simulink model "amk_sim_model"  (R2022b)
settings: Solver=FixedStepAuto  StartTime=0.0  StopTime=4  FixedStep=1e-6  MaxStep=1e-5  MinStep=1e-6  RelTol=1e-3
values from neighbouring files (symbols this model uses):
  a_fw = log(9)/trfw    [amk_sim.m]    (also in amk_sim_2.m)
  ac = log(9)/tr    [amk_sim.m]    (also in amk_sim_2.m)
  ar_max = 1500    [amk_sim_2.m]
  as = log(9)/trs    [amk_sim.m]    (also in amk_sim_2.m)
  ba = 2*k^2*(as*J - 0)/(np^2*psi)    [amk_sim.m]    (also in amk_sim_2.m = 2*k^2*(as*J - bm)/(np^2*psi))
  bm = 0.02    [amk_sim.m]    (also in amk_sim_2.m = 0.008)
  I_base = 85.7    [amk_sim.m]    (also in amk_sim_2.m)
  I_max = 85.7    [amk_sim.m]    (also in amk_sim_2.m)
  Icon = 33.5    [amk_sim.m]    (also in amk_sim_2.m)
  Imax_interval = 1.24    [amk_sim.m]    (also in amk_sim_2.m = 5)
  Ipeak = 85.7    [amk_sim.m]    (also in amk_sim_2.m = 87.5)
  J = 2.5*(2.74e-4)    (= 0.000685)    [amk_sim.m]    (also in amk_sim_2.m = 0.000528)
  k = 1    [amk_sim.m]    (also in amk_sim_2.m)
  ki_ar = 0.2    [amk_sim_2.m]
  ki_s = 2*k^2*as^2*J/(np^2*psi)    [amk_sim.m]    (also in amk_sim_2.m)
  kp_ar = 1e-5    (= 1e-05)    [amk_sim_2.m]
  kp_s = 2*k^2*as*J/(np^2*psi)    [amk_sim.m]    (also in amk_sim_2.m)
  Ld = Ldm    (= 0.0004)    [amk_sim.m]    (also in amk_sim_2.m = 0.00012)
  Lq = Lqm    (= 0.00052)    [amk_sim.m]    (also in amk_sim_2.m = 0.00024)
  max_temp = 140    [amk_sim.m]    (also in amk_sim_2.m)
  np = 5    [amk_sim.m]    (also in amk_sim_2.m)
  Peak_power = 45000    [amk_sim.m]    (also in amk_sim_2.m = 50000)
  Peak_regen = -15000    [amk_sim.m]    (also in amk_sim_2.m = -1500000)
  psi = 0.047    [amk_sim.m]    (also in amk_sim_2.m = 0.05077789)
  rpm_nom = 20000    [amk_sim.m]    (also in amk_sim_2.m = 12000)
  Rs = 202.5e-3    (= 0.2025)    [amk_sim.m]    (also in amk_sim_2.m)
  sample_time = 1e-4    (= 0.0001)    [amk_sim.m]    (also in amk_sim_2.m = 1e-06)
  temp_threshold = 100    [amk_sim.m]    (also in amk_sim_2.m)
  u_dc = 550    [amk_sim.m]    (also in amk_sim_2.m)
  u_nom = u_dc*k    (= 550)    [amk_sim.m]    (also in amk_sim_2.m)
undefined symbols (not defined in the file or in its folder): sigbuilder_block
libraries: simulink x3
(part 1 of 5)
settings Model: Creator=Vaggelis  LastModifiedBy=alexa
settings SolverCC: ZeroCrossAlgorithm=Adaptive
settings OptimizationCC: ReuseModelBlockBuffer=on
settings DebuggingCC: IgnoredZcDiagnostic=none  UnconnectedInputMsg=warning  UnconnectedOutputMsg=warning  UnconnectedLineMsg=warning  ArithmeticOperatorsInVariantConditions=warning
settings ModelReferenceCC: EnableRefExpFcnMdlSchedulingChecks=on  ModelReferenceMinAlgLoopOccurrences=on
settings SFSimCC: CustomCodeUndefinedFunction=UseInterfaceOnly
settings RTWCC: DLArmComputeVersion=19.05

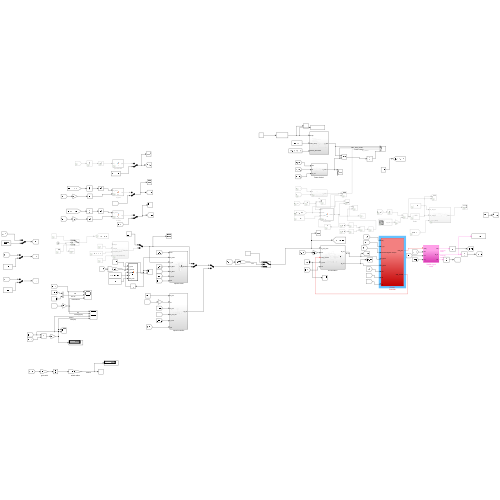
[thumbnail: Simulink's stored preview of the top-level diagram]
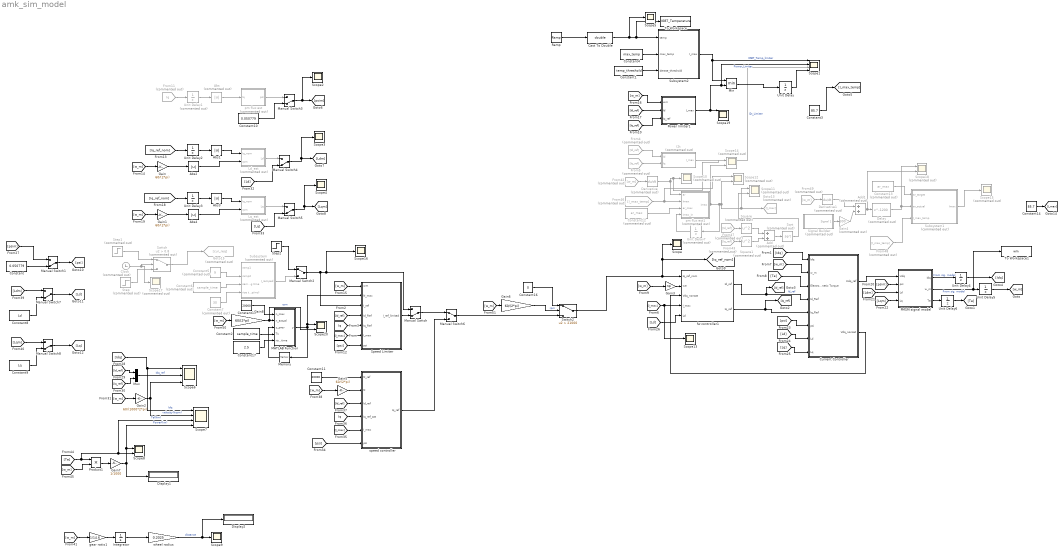
== system amk_sim_model ==
  Abs : Abs  Commented=on  SaturateOnIntegerOverflow=off
  Abs{1..4} (4 alike) : Abs  SaturateOnIntegerOverflow=off
  Add : Sum  Commented=on
  Add1 : Sum  Commented=on
  Cast To Double : DataTypeConversion  OutDataTypeStr=double  SaturateOnIntegerOverflow=off  RndMeth=Floor
  Clock : Clock  Commented=on
  Constant : Constant  Value=0.050779
  Constant1 : Constant  Value=temp_threshold
  Constant10 : Constant  Value=0.050779
  Constant11 : Constant  Value=20000
  Constant12 : Constant  Commented=on  Value=ar_max
  Constant13 : Constant  Commented=on  Value=ar_max
  Constant14 : Constant  Value=85.7
  Constant15 : Constant  Value=20000
  Constant16 : Constant  Value=0
  Constant17 : Constant  Value=2.5
  Constant2 : Constant  Value=sample_time
  Constant3 : Constant  Value=85.7
  Constant4 : Constant  Value=max_temp
  Constant5 : Constant  Commented=on  Value=9
  Constant6 : Constant  Commented=on  Value=sample_time
  Constant7 : Constant  Commented=on  Value=30
  Constant8 : Constant  Value=Ld
  Constant9 : Constant  Value=Lq
  Current Controller : Subsystem
  Delay : Delay  Commented=on  DelayLength=1200  InitialCondition=0  UseCircularBuffer=on
  Derivative : Derivative  Commented=on
  Derivative1 : Derivative  Commented=on
  Display1 : Display
  Display2 : Display
  From11 : From  Commented=on  GotoTag=Iq  TagVisibility=global
  From4 : From  Commented=on  GotoTag=Id_ref
  From42 : From  Commented=on  GotoTag=w_m
  From43 : From  Commented=on  GotoTag=Iq_ref
  From46 : From  Commented=on  GotoTag=I_max_temp
  From47 : From  Commented=on  GotoTag=Id_ref
  From48 : From  Commented=on  GotoTag=I_max_temp
  From49 : From  Commented=on  GotoTag=w_m
  From5 : From  Commented=on  GotoTag=Iq_ref
  Gain{,1,5..6,8} (5 alike) : Gain  Gain=60/(2*pi)
  Gain2 : Gain  Gain=60/(1000*2*pi)
  Gain3 : Gain  Gain=np
  Gain4 : Gain  Commented=on  Gain=300
  Gain7 : Gain  Gain=1/1000
  Goto13 : Goto  Commented=on  GotoTag=I_max
  Goto15 : Goto  Commented=on  GotoTag=cur_req
  I2t : Subsystem  Commented=on
  Integrator : Integrator
  Ld_est : MATLAB Function  Commented=on  TreatAsAtomicUnit=on
  Lq_est : MATLAB Function  Commented=on  TreatAsAtomicUnit=on
  MATLAB Function : MATLAB Function  TreatAsAtomicUnit=on
  Manual Switch{,1,3..5,7..8} (7 alike) : ManualSwitch  CurrentSetting=0
  Manual Switch2 : ManualSwitch
  Manual Switch6 : ManualSwitch
  Memory : Memory
  Min : MinMax  Inputs=2
  Mux : Mux  Inputs=2
  PMSM signal model : Subsystem
  Power limiter1 : Subsystem
  Product1 : Product
  Ramp : simulink/Sources/Ramp  slope=1  start=0  InitialOutput=30
  Scope{,2..5,9,13,16} (8 alike) : Scope
  Scope1 : Scope  NumInputPorts=4
  Scope10 : Scope  Commented=on
  Scope{11..12,14,18} (4 alike) : Scope  Commented=on  NumInputPorts=2
  Scope15 : Scope  Commented=on
  Scope17 : Scope  Commented=on
  Scope19 : Scope  NumInputPorts=4
  Scope20 : Scope  NumInputPorts=2
  Scope6 : Scope  NumInputPorts=3
  Scope7 : Scope  NumInputPorts=4
  Scope8 : Scope  NumInputPorts=2
  Signal Builder : Subsystem  Tag=STV Subsys  Commented=on  LoadFcn=sigbuilder_block('load');  StartFcn=sigbuilder_block('start');  StopFcn=sigbuilder_block('stop');  ClipboardFcn=sigbuilder_block('clipboard');  mask(Sigbuilder block){tuvar=[0:10]}
      mask help: Simulink:masks:SigbuilderBlock_MD
      mask init:
      | if ~strcmp(get_param(bdroot(gcbh),'SimulationStatus'),'stopped') tuvar = sigbuilder_block('maskInit'); end
      settings: CopyFcn=sigbuilder_block('copy');  DeleteFcn=sigbuilder_block('delete');  ModelCloseFcn=sigbuilder_block('modelClose');  PreSaveFcn=sigbuilder_block('preSave');  PauseFcn=sigbuilder_block('pause');  ContinueFcn=sigbuilder_block('continue');  NameChangeFcn=sigbuilder_block('namechange');  OpenFcn=sigbuilder_block('open',[437.6 199.2 550.4 400 ]);  CloseFcn=sigbuilder_block('close');
      mask Display: plot(0, 0, 100, 100,[2, 2, 32, 32, 2], [68, 8, 8, 68, 68],[32, 2], [38, 38], [32, 19, 2],[53, 60, 44], [32, 17, 17, 2],[16, 16, 31, 31]);txt = getActiveGroup(gcbh);text(2, 100, txt,'verticalAlignment', 'top');
  Speed Limiter : Subsystem
  Sqrt : Sqrt  Commented=on
  Square : Math  Commented=on  Operator=square
  Square1 : Math  Commented=on  Operator=square
  Step : Step  Commented=on  Time=0.3  After=90  SampleTime=0
  Step1 : Step  Commented=on  After=90  SampleTime=0
  Step2 : Step  Time=0.5  Before=90  After=90  SampleTime=0
  Subsystem : Subsystem  Commented=on
  Subsystem1 : Subsystem  Commented=on
  Subsystem2 : Subsystem
  Switch : Switch  Commented=on  Criteria=u2 > Threshold  Threshold=0.8  SaturateOnIntegerOverflow=off  InputSameDT=off
  Switch2 : Switch  Criteria=u2 > Threshold  Threshold=21000  SaturateOnIntegerOverflow=off  InputSameDT=off
  To Workspace : ToWorkspace  VariableName=IGBT_Temperature  SampleTime=-1
  To Workspace1 : ToWorkspace  VariableName=wm  SampleTime=-1
  Unit Delay{,2..6} (6 alike) : UnitDelay  SampleTime=-1  HasFrameUpgradeWarning=on
  Unit Delay1 : UnitDelay  Commented=on  SampleTime=-1  HasFrameUpgradeWarning=on
  Unit Delay7 : UnitDelay  Commented=on  SampleTime=-1  HasFrameUpgradeWarning=on
  fw controller1 : Subsystem
  gear ratio1 : Gain  Gain=1/14.6
  pm flux est : MATLAB Function  Commented=on  TreatAsAtomicUnit=on
  pm flux est1 : MATLAB Function  Commented=on  TreatAsAtomicUnit=on
  speed controller : Subsystem
  wheel radius : Gain  Gain=0.2025
  wires:
  PMSM signal model/2("w_m ") -> To Workspace1/1, Unit Delay5/1  "From sig. model"
  Gain3/1 -> fw controller1/2(we)
  Current Controller/2(Vdq_nonsat) -> fw controller1/3(Vdq_nonsat)
  PMSM signal model/1(Idq) -> Unit Delay4/1  "From sig. model"
  [Idq] -> Current Controller/1(Idq)
  [w_m] -> Current Controller/2(w_m)
  [Te] -> Current Controller/3(Electromagnetic Torque)
  [w_m] -> Power limiter1/1(wm)
  [Id_ref] -> Power limiter1/2(Id)
  Current Controller/1("Udq_ref ") -> PMSM signal model/1(Udq)
  Constant5/1 -> Subsystem/2(ramp2)
  Constant6/1 -> Subsystem/3(sampling time)
  Constant7/1 -> Subsystem/4(rise time (Amp/ms))
  Constant4/1 -> Subsystem2/2(max_temp)
  Ramp/1 -> Cast To Double/1
  Cast To Double/1 -> Subsystem2/1(temp), To Workspace/1, Scope5/1
  fw controller1/1(Id_ref) -> Current Controller/4(Id_Ref), [Id_ref]  "Id_ref"
  From4/1 -> I2t/1(Id)
  From5/1 -> I2t/2(Iq)
  Subsystem2/1(I_max) -> Min/1, Scope1/1  "IGBT_Temp_limiter"
  Power limiter1/1(I_max) -> Scope1/2, Min/2, Scope19/1  "Power_Limiter"
  I2t/1(I_max) -> Scope1/3  "I2t_Limiter"
  [I_max] -> Speed Limiter/6(I_max)
  Unit Delay/1 -> Scope1/4
  [Iq_ref] -> Power limiter1/3(Iq_ref)
  Constant1/1 -> Subsystem2/3(derate_threshold)
  [I_max] -> Scope13/1, fw controller1/4(I_max)
  [Id_ref] -> Speed Limiter/4(Id_Ref)
  [Iq] -> Speed Limiter/5(Iq_Ref)
  [w_m] -> Speed Limiter/1(wm)
  [w_m] -> Gain3/1
  PMSM signal model/3("Te ") -> Unit Delay6/1
  Abs/1 -> pm flux est/1(Iq)
  From11/1 -> Unit Delay1/1
  [psi] -> Speed Limiter/7(psi)
  Unit Delay1/1 -> Abs/1
  Unit Delay2/1 -> Abs1/1
  [Iq_ref_nom] -> Unit Delay2/1
  Abs1/1 -> Ld_est/1(Iq_nom)
  [w_m] -> Gain/1
  Gain/1 -> Abs2/1
  Abs2/1 -> Ld_est/2(rpm)
  Abs4/1 -> Lq_est/2(rpm)
  Gain1/1 -> Abs4/1
  [w_m] -> Gain1/1
  Abs3/1 -> Lq_est/1(Iq_nom)
  [Iq_ref_nom] -> Unit Delay3/1
  Unit Delay3/1 -> Abs3/1
  [psim] -> PMSM signal model/2(psi)
  [Ldm] -> PMSM signal model/3(Ld)
  [Lqm] -> PMSM signal model/4(Lq)
  [psi] -> Current Controller/6(psi)
  [Ld] -> Current Controller/7(Ld)
  [Lq] -> Current Controller/8(Lq)
  [Ld] -> fw controller1/5(Ld)
  Speed Limiter/1(I_ref_limited) -> Manual Switch/2
  Unit Delay4/1 -> [Idq]
  Unit Delay5/1 -> [w_m]
  Unit Delay6/1 -> [Te]
  Manual Switch1/1 -> [psi]
  Constant/1 -> Manual Switch1/2
  [psim] -> Manual Switch1/1
  [Id_ref] -> Mux/1
  [Iq_ref] -> Mux/2
  Mux/1 -> Scope6/2  "Idq_ref"
  [Idq] -> Scope7/1, Scope6/1  "Idq"
  [w_m] -> Gain2/1
  Gain2/1 -> Scope6/3, Scope7/2  "velocity(krpm)"
  Subsystem/1(I_ramped) -> Manual Switch2/2
  Manual Switch2/1 -> Speed Limiter/3(I_ref), Scope16/1, Manual Switch/1
  pm flux est/1(psi) -> Manual Switch3/1
  Manual Switch3/1 -> Scope2/1, [psim]
  Constant10/1 -> Manual Switch3/2
  Ld_est/1(Ld) -> Manual Switch4/1
  Manual Switch4/1 -> [Ldm], Scope3/1
  [Ld] -> Manual Switch4/2
  Lq_est/1(Lq) -> Manual Switch5/1
  Manual Switch5/1 -> Scope4/1, [Lqm]
  [Lq] -> Manual Switch5/2
  speed controller/1(Iq_ref) -> Manual Switch6/2
  Constant11/1 -> speed controller/1(N_ref)
  [Iq] -> speed controller/4(Iq_ref_sat)
  [w_m] -> Gain5/1
  Gain5/1 -> speed controller/2(N)
  [Id_ref] -> speed controller/3(Id_ref)
  [psi] -> speed controller/6(psi)
  [I_max] -> speed controller/5(I_max)
  Manual Switch/1 -> Manual Switch6/1
  Manual Switch7/1 -> [Ld]
  Constant8/1 -> Manual Switch7/2
  Manual Switch8/1 -> [Lq]
  Constant9/1 -> Manual Switch8/2
  [Ldm] -> Manual Switch7/1
  [Lqm] -> Manual Switch8/1
  Gain7/1 -> Scope7/4, Scope8/1, Display1/1  "Power(kw)"
  Product1/1 -> Gain7/1
  [w_m] -> Product1/2
  [Te] -> Product1/1, Scope7/3, Scope8/2  "Te(Nm)"
  [w_m] -> gear ratio1/1
  Integrator/1 -> wheel radius/1
  wheel radius/1 -> Display2/1, Scope9/1  "distance"
  gear ratio1/1 -> Integrator/1
  Derivative/1 -> pm flux est1/1(ar), Scope14/1, Scope10/1
  From42/1 -> Derivative/1
  Min/1 -> Unit Delay/1
  From46/1 -> Scope12/1, pm flux est1/2(Imax)
  Constant12/1 -> pm flux est1/3(ar_max)
  Unit Delay7/1 -> pm flux est1/4(imax_in)
  From47/1 -> Square/1
  From43/1 -> Square1/1
  Square/1 -> Add/1
  Square1/1 -> Add/2
  Add/1 -> Sqrt/1
  Sqrt/1 -> Scope11/2
  pm flux est1/1(imax) -> Scope14/2, Unit Delay7/1, Scope12/2, Goto13/1, Scope11/1
  Constant13/1 -> Subsystem1/1(ar_target)
  From49/1 -> Derivative1/1
  Switch/1 -> Goto15/1
  Clock/1 -> Scope17/1, Switch/2
  Step/1 -> Switch/3
  Step1/1 -> Switch/1
  From48/1 -> Subsystem1/3(I_max_temp)
  Derivative1/1 -> Add1/1
  Signal Builder/1(Signal 1) -> Gain4/1
  Gain4/1 -> Add1/2
  Add1/1 -> Scope18/2, Delay/1
  Delay/1 -> Scope18/1, Subsystem1/2(ar_actual)
  Constant3/1 -> [I_max_temp]
  Step2/1 -> Manual Switch2/1
  Subsystem1/1(Imax) -> Scope15/1
  Constant14/1 -> [I_max]
  fw controller1/2(Iq_ref) -> [Iq_ref], Current Controller/5(Iq_Ref)
  Gain6/1 -> Switch2/2  "rpm"
  [w_m] -> Gain6/1
  Constant16/1 -> Switch2/1
  Manual Switch6/1 -> Switch2/3
  Switch2/1 -> Scope/1, [Iq_ref_nom], fw controller1/1(Iq_ref_nom)
  Constant15/1 -> MATLAB Function/1(n_max)
  MATLAB Function/1(y) -> Speed Limiter/2(N_max), Scope20/1, Memory/1
  Constant2/1 -> MATLAB Function/4(Ts)
  Constant17/1 -> MATLAB Function/5(rise_time)
  Memory/1 -> MATLAB Function/3(y_prev)
  [w_m] -> Gain8/1
  Gain8/1 -> Scope20/2, MATLAB Function/2(n_actual)  "rpm"

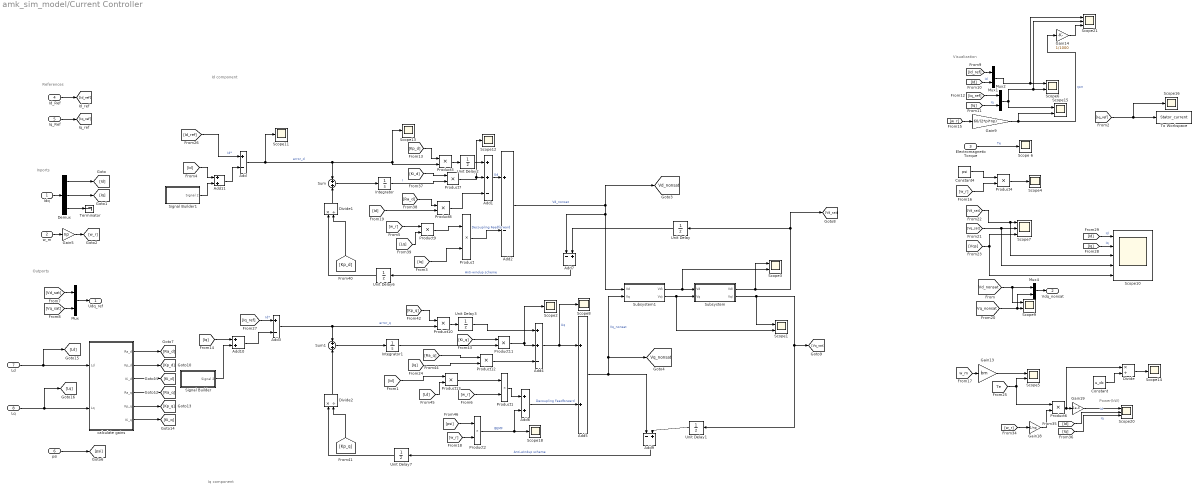
== system amk_sim_model/Current Controller ==
  note: References
  note: Id component
  note: Iq component
  note: Inports
  note: Outports
  note: Visualization
  note: Power(kW)
  Idq : Inport
  w_m : Inport  Port=2
  Electromagnetic Torque : Inport  Port=3
  Id_Ref : Inport  Port=4
  Iq_Ref : Inport  Port=5
  psi : Inport  Port=6
  Ld : Inport  Port=7
  Lq : Inport  Port=8
  Add : Sum  Inputs=+-
  Add1 : Sum  Inputs=++-
  Add{5..6,10..11} (4 alike) : Sum
  Add2 : Sum  Inputs=+-
  Add3 : Sum  Inputs=+-
  Add4 : Sum  Inputs=++-
  Add7 : Sum  Inputs=-+
  Add9 : Sum  Inputs=-+
  Constant : Constant  Value=u_dc
  Constant4 : Constant  Value=psi
  Demux : Demux  Outputs=3
  Divide : Product  Inputs=*/
  Divide1 : Product  Inputs=*/
  Divide2 : Product  Inputs=*/
  Gain13 : Gain  Gain=bm
  Gain14 : Gain  Gain=1/1000
  Gain18 : Gain  Gain=1/np
  Gain19 : Gain  Gain=1e-3
  Gain5 : Gain  Gain=np
  Gain9 : Gain  Gain=60/(2*pi*np)
  Integrator : Integrator
  Integrator1 : Integrator
  Mux{,1..2,4} (4 alike) : Mux  Inputs=2
  Product{,1..4,6..13} (13 alike) : Product
  Scope 6 : Scope
  Scope{1,3,5..6,9,15} (6 alike) : Scope  NumInputPorts=2
  Scope10 : Scope  NumInputPorts=5
  Scope{2,4,8,11..14,16,18} (9 alike) : Scope
  Scope20 : Scope  NumInputPorts=3
  Scope21 : Scope  NumInputPorts=3
  Scope7 : Scope  NumInputPorts=3
  Signal Builder : Subsystem  Tag=STV Subsys  LoadFcn=sigbuilder_block('load');  StartFcn=sigbuilder_block('start');  StopFcn=sigbuilder_block('stop');  ClipboardFcn=sigbuilder_block('clipboard');  mask(Sigbuilder block){tuvar=[0:10]}
      mask help: Simulink:masks:SigbuilderBlock_MD
      mask init:
      | if ~strcmp(get_param(bdroot(gcbh),'SimulationStatus'),'stopped') tuvar = sigbuilder_block('maskInit'); end
      settings: CopyFcn=sigbuilder_block('copy');  DeleteFcn=sigbuilder_block('delete');  ModelCloseFcn=sigbuilder_block('modelClose');  PreSaveFcn=sigbuilder_block('preSave');  PauseFcn=sigbuilder_block('pause');  ContinueFcn=sigbuilder_block('continue');  NameChangeFcn=sigbuilder_block('namechange');  OpenFcn=sigbuilder_block('open',[437.6 199.2 550.4 400 ]);  CloseFcn=sigbuilder_block('close');
      mask Display: plot(0, 0, 100, 100,[2, 2, 32, 32, 2], [68, 8, 8, 68, 68],[32, 2], [38, 38], [32, 19, 2],[53, 60, 44], [32, 17, 17, 2],[16, 16, 31, 31]);txt = getActiveGroup(gcbh);text(2, 100, txt,'verticalAlignment', 'top');
  Signal Builder1 : Subsystem  Tag=STV Subsys  LoadFcn=sigbuilder_block('load');  StartFcn=sigbuilder_block('start');  StopFcn=sigbuilder_block('stop');  ClipboardFcn=sigbuilder_block('clipboard');  mask(Sigbuilder block){tuvar=[0:10]}
      mask help: Simulink:masks:SigbuilderBlock_MD
      mask init:
      | if ~strcmp(get_param(bdroot(gcbh),'SimulationStatus'),'stopped') tuvar = sigbuilder_block('maskInit'); end
      settings: CopyFcn=sigbuilder_block('copy');  DeleteFcn=sigbuilder_block('delete');  ModelCloseFcn=sigbuilder_block('modelClose');  PreSaveFcn=sigbuilder_block('preSave');  PauseFcn=sigbuilder_block('pause');  ContinueFcn=sigbuilder_block('continue');  NameChangeFcn=sigbuilder_block('namechange');  OpenFcn=sigbuilder_block('open',[437.6 199.2 550.4 400 ]);  CloseFcn=sigbuilder_block('close');
      mask Display: plot(0, 0, 100, 100,[2, 2, 32, 32, 2], [68, 8, 8, 68, 68],[32, 2], [38, 38], [32, 19, 2],[53, 60, 44], [32, 17, 17, 2],[16, 16, 31, 31]);txt = getActiveGroup(gcbh);text(2, 100, txt,'verticalAlignment', 'top');
  Subsystem : Subsystem
  Subsystem1 : Subsystem
  Sum : Sum
  Sum1 : Sum
  Terminator : Terminator
  To Workspace : ToWorkspace  VariableName=Stator_current  SampleTime=-1
  Unit Delay{,1..3,6..7} (6 alike) : UnitDelay  SampleTime=-1  HasFrameUpgradeWarning=on
  calculate gains : Subsystem
  "Udq_ref " : Outport  VectorParamsAs1DForOutWhenUnconnected=off
  Vdq_nonsat : Outport  Port=2
  tag scope: Vd_nonsat=global, Vq_nonsat=global
  wires:
  Product11/1 -> Add4/2, Scope2/1
  Add4/1 -> Scope8/1, Add5/1  "Uq"
  Add1/1 -> Add2/1  "Ud"
  Product9/1 -> Product/1
  Product10/1 -> Unit Delay3/1
  Product3/1 -> Unit Delay2/1
  [w_r] -> Product1/2
  Product13/1 -> Product1/1
  Idq/1 -> Demux/1
  Product/1 -> Add2/2  "Decoupling Feedforward"
  Divide1/1 -> Sum/2
  Add2/1 -> [Vd_nonsat], Subsystem1/1(Vd), Add7/1  "Vd_nonsat"
  Add7/1 -> Unit Delay6/1  "Anti-windup scheme"
  Add5/1 -> Add9/1, Subsystem1/2(Vq), [Vq_nonsat]  "Vq_nonsat"
  Divide2/1 -> Sum1/2
  Add9/1 -> Unit Delay7/1  "Anti-windup scheme"
  Demux/1 -> [Id]
  Demux/2 -> [Iq]
  Demux/3 -> Terminator/1
  w_m/1 -> Gain5/1
  Gain5/1 -> [w_r]
  [Vd_sat] -> Mux/1
  [Vq_sat] -> Mux/2
  Mux/1 -> "Udq_ref "/1
  Mux1/1 -> Scope21/1, Scope6/1
  [Id_ref] -> Mux1/1
  [Id] -> Mux1/2  "Id"
  [Iq_ref] -> Mux2/1
  [Iq] -> Mux2/2  "Iq"
  [w_r] -> Gain9/1
  Gain9/1 -> Scope15/2, Gain14/1  "rpm"
  [psi] -> Product2/1
  Product1/1 -> Add6/1
  Add6/1 -> Add5/2  "Decoupling Feedforward"
  Add/1 -> Product3/2, Scope13/1, Sum/1, Scope11/1  "error_d"
  Add3/1 -> Product10/2, Sum1/1  "error_q"
  Product7/1 -> Scope12/1, Add1/2
  [Vd_nonsat] -> Scope9/1, Mux4/1
  [Vq_nonsat] -> Mux4/2, Scope9/2
  [Vd_sat] -> Scope10/3, Scope7/1
  [Vq_sat] -> Scope10/4, Scope7/2
  [Vqs] -> Scope7/3, Scope10/5
  [w_r] -> Product4/2
  Constant4/1 -> Product4/1
  Product4/1 -> Scope4/1
  Id_Ref/1 -> [Id_ref]
  Iq_Ref/1 -> [Iq_ref]
  Gain13/1 -> Scope5/1
  [Te] -> Product6/1, Scope5/2
  [w_m] -> Gain13/1
  Mux2/1 -> Scope21/2, Scope6/2, Scope15/1
  [Iq] -> Scope10/2  "Iq"
  [Id] -> Scope10/1  "Id"
  [Id_ref] -> Add/1  "Id*"
  [w_r] -> Product2/2
  Product2/1 -> Scope18/1, Add6/2  "BEMF"
  Mux4/1 -> Vdq_nonsat/1
  [Iq_ref] -> Add3/1  "Id*"
  Gain19/1 -> Scope20/1
  [Iq] -> Scope20/3  "Iq"
  [Id] -> Scope20/2  "Id"
  Gain18/1 -> Product6/2
  Product6/1 -> Divide/1, Gain19/1
  [w_r] -> Gain18/1
  Product12/1 -> Add4/3
  Product8/1 -> Add1/3
  Constant/1 -> Divide/2
  Divide/1 -> Scope14/1
  [Id] -> Product8/2
  [Iq] -> Product/2
  [Iq_ref] -> To Workspace/1, Scope16/1
  Electromagnetic Torque/1 -> Scope 6/1  "Te"
  Unit Delay/1 -> Add7/2
  Unit Delay1/1 -> Add9/2
  Gain14/1 -> Scope21/3
  [Kp_d] -> Product3/1
  Integrator/1 -> Product7/2  "I"
  [Ki_d] -> Product7/1
  [Ra_d] -> Product8/1
  [w_r] -> Product9/1
  [Lq] -> Product9/2
  [Kp_q] -> Product10/1
  [Ki_q] -> Product11/1
  Integrator1/1 -> Product11/2
  [Iq] -> Product12/2
  [Ra_q] -> Product12/1
  [Ld] -> Product13/2
  [Id] -> Product13/1
  Ld/1 -> [Ld], calculate gains/1(Ld)
  Lq/1 -> [Lq], calculate gains/2(Lq)
  psi/1 -> [psi]
  calculate gains/1(Ra_d) -> [Ra_d]
  calculate gains/2(Kp_d) -> [Kp_d]
  calculate gains/3(Ki_d) -> [Ki_d]
  calculate gains/4(Ra_q) -> [Ra_q]
  calculate gains/5(Kp_q) -> [Kp_q]
  calculate gains/6(Ki_q) -> [Ki_q]
  Unit Delay2/1 -> Add1/1
  Unit Delay3/1 -> Add4/1
  Sum/1 -> Integrator/1
  Sum1/1 -> Integrator1/1
  Unit Delay6/1 -> Divide1/1
  Unit Delay7/1 -> Divide2/1
  [Kp_d] -> Divide1/2
  [Kp_q] -> Divide2/2
  Signal Builder/1(Signal 2) -> Add10/2
  Signal Builder1/1(Signal 2) -> Add11/2
  Subsystem1/2(Vq\) -> Scope1/2, Subsystem/2(Vq)
  Subsystem1/1(Vd\) -> Scope3/2, Subsystem/1(Vd)
  Subsystem/1(Vd\) -> Scope3/1, [Vd_sat], Unit Delay/1
  Subsystem/2(Vq\) -> Scope1/1, Unit Delay1/1, [Vq_sat]
  [Iq] -> Add10/1
  Add10/1 -> Add3/2
  [Id] -> Add11/1
  Add11/1 -> Add/2

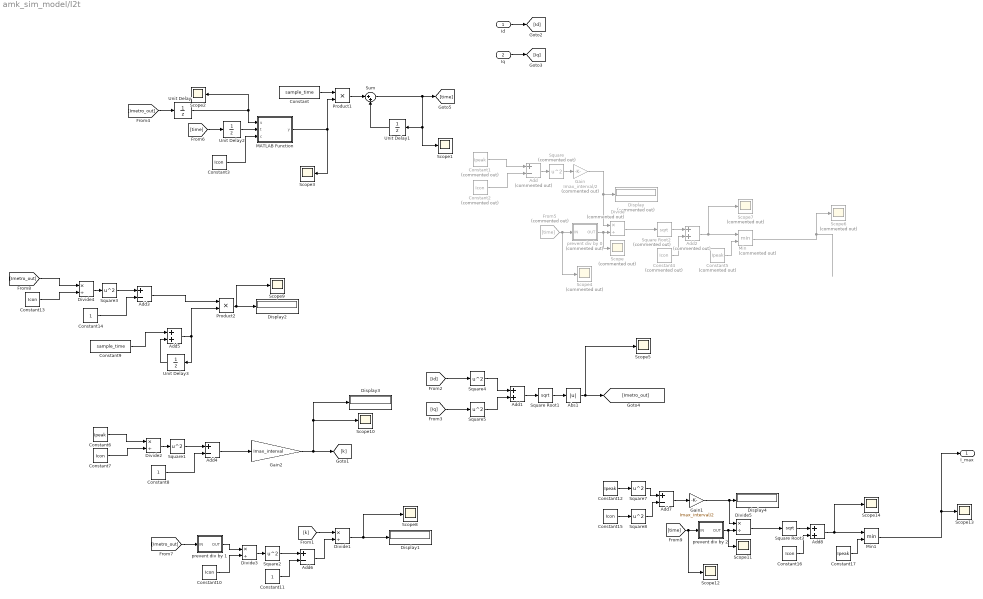
== system amk_sim_model/I2t ==
  Id : Inport
  Iq : Inport  Port=2
  Abs1 : Abs  SaturateOnIntegerOverflow=off
  Add : Sum  Commented=on  Inputs=+-
  Add1 : Sum
  Add2 : Sum  Commented=on
  Add{3..4,6..7} (4 alike) : Sum  Inputs=+-
  Add5 : Sum
  Add8 : Sum
  Constant : Constant  Value=sample_time
  Constant1 : Constant  Commented=on  Value=Ipeak
  Constant{3,7,10,13,15..16} (6 alike) : Constant  Value=Icon
  Constant11 : Constant
  Constant12 : Constant  Value=Ipeak
  Constant14 : Constant
  Constant17 : Constant  Value=Ipeak
  Constant2 : Constant  Commented=on  Value=Icon
  Constant4 : Constant  Commented=on  Value=Icon
  Constant5 : Constant  Commented=on  Value=Ipeak
  Constant6 : Constant  Value=Ipeak
  Constant8 : Constant
  Constant9 : Constant  Value=sample_time
  Display : Display  Commented=on
  Display{1..4} (4 alike) : Display
  Divide : Product  Commented=on  Inputs=*/
  Divide{1..5} (5 alike) : Product  Inputs=*/
  From5 : From  Commented=on  GotoTag=time
  Gain : Gain  Commented=on  Gain=Imax_interval/2
  Gain1 : Gain  Gain=Imax_interval/2
  Gain2 : Gain  Gain=Imax_interval
  MATLAB Function : MATLAB Function  TreatAsAtomicUnit=on
  Min : MinMax  Commented=on  Inputs=2
  Min1 : MinMax  Inputs=2
  Product1 : Product
  Product2 : Product
  Scope{,4,6..7} (4 alike) : Scope  Commented=on
  Scope{1..3,5,8..14} (11 alike) : Scope
  Square : Math  Commented=on  Operator=square
  Square Root1 : Sqrt
  Square Root2 : Sqrt  Commented=on
  Square Root3 : Sqrt
  Square{1..5,7..8} (7 alike) : Math  Operator=square
  Sum : Sum  Inputs=|++
  Unit Delay{,1..3} (4 alike) : UnitDelay  SampleTime=-1  HasFrameUpgradeWarning=on
  prevent div by 0 : Subsystem  Commented=on
  prevent div by 1 : Subsystem
  prevent div by 2 : Subsystem
  I_max : Outport
  wires:
  Iq/1 -> [Iq]
  Id/1 -> [Id]
  Divide/1 -> Square Root2/1
  prevent div by 0/1(OUT) -> Scope/1, Divide/2
  From5/1 -> Scope4/1, prevent div by 0/1(IN)
  Sum/1 -> Unit Delay1/1, Scope1/1, [time]
  [Imetro_out] -> Unit Delay/1
  [time] -> Unit Delay2/1
  Unit Delay1/1 -> Sum/2
  Add1/1 -> Square Root1/1
  Square5/1 -> Add1/2
  Square4/1 -> Add1/1
  Square Root1/1 -> Abs1/1
  Constant/1 -> Product1/1
  Product1/1 -> Sum/1
  MATLAB Function/1(y) -> Product1/2, Scope3/1
  Constant3/1 -> MATLAB Function/3(c)
  Abs1/1 -> Scope5/1, [Imetro_out]
  Min/1 -> Scope6/1
  Unit Delay/1 -> MATLAB Function/1(u), Scope2/1
  Unit Delay2/1 -> MATLAB Function/2(t)
  Gain/1 -> Display/1, Divide/1
  Constant1/1 -> Add/1
  Add/1 -> Square/1
  Constant2/1 -> Add/2
  Square Root2/1 -> Add2/1
  Add2/1 -> Min/1, Scope7/1
  Constant4/1 -> Add2/2
  Square/1 -> Gain/1
  [Id] -> Square4/1
  [Iq] -> Square5/1
  Constant5/1 -> Min/2
  Constant7/1 -> Divide2/2
  Divide2/1 -> Square1/1
  Constant6/1 -> Divide2/1
  Square1/1 -> Add4/1
  Constant8/1 -> Add4/2
  Add4/1 -> Gain2/1
  Constant11/1 -> Add6/2
  Square2/1 -> Add6/1
  [Imetro_out] -> prevent div by 1/1(IN)
  Divide3/1 -> Square2/1
  Constant10/1 -> Divide3/2
  prevent div by 1/1(OUT) -> Divide3/1
  Add6/1 -> Divide1/2
  Divide1/1 -> Scope8/1, Display1/1
  [k] -> Divide1/1
  Gain2/1 -> [k], Display3/1, Scope10/1
  Constant14/1 -> Add3/2
  Square3/1 -> Add3/1
  [Imetro_out] -> Divide4/1
  Divide4/1 -> Square3/1
  Constant13/1 -> Divide4/2
  Unit Delay3/1 -> Add5/2
  Add5/1 -> Unit Delay3/1, Product2/2
  Constant9/1 -> Add5/1
  Add3/1 -> Product2/1
  Product2/1 -> Scope9/1, Display2/1
  Constant17/1 -> Min1/2
  Add7/1 -> Gain1/1
  Constant16/1 -> Add8/2
  Add8/1 -> Scope14/1, Min1/1
  Square Root3/1 -> Add8/1
  Gain1/1 -> Display4/1, Divide5/1
  Min1/1 -> I_max/1, Scope13/1
  [time] -> prevent div by 2/1(IN), Scope12/1
  prevent div by 2/1(OUT) -> Divide5/2, Scope11/1
  Divide5/1 -> Square Root3/1
  Constant12/1 -> Square7/1
  Constant15/1 -> Square8/1
  Square7/1 -> Add7/1
  Square8/1 -> Add7/2

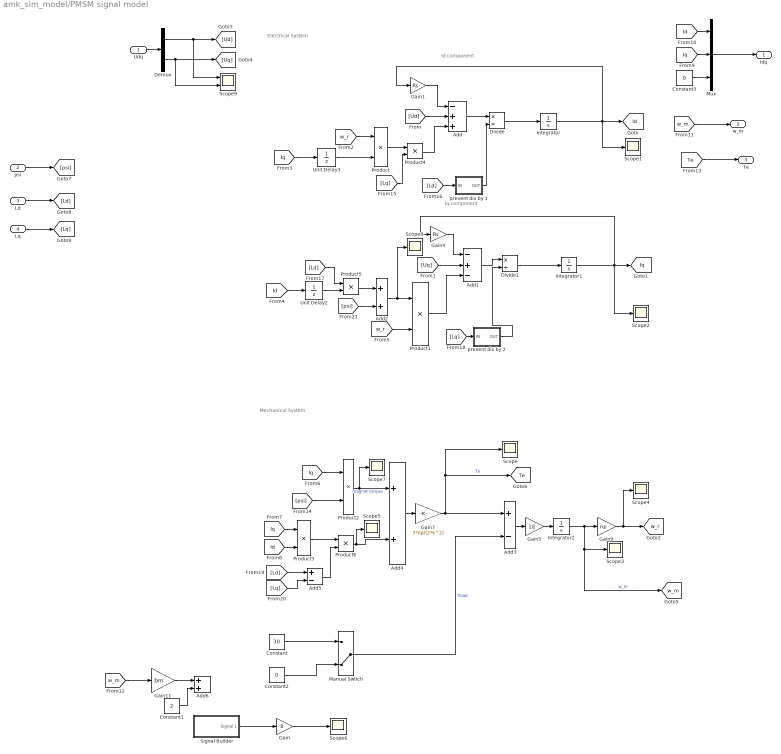
== system amk_sim_model/PMSM signal model ==
  note: Electrical System
  note: Id component
  note: Iq component
  note: Mechanical System
  Udq : Inport
  psi : Inport  Port=2
  Ld : Inport  Port=3
  Lq : Inport  Port=4
  Add : Sum  Inputs=-++
  Add1 : Sum  Inputs=-+-
  Add2 : Sum
  Add3 : Sum  Inputs=+-
  Add4 : Sum
  Add5 : Sum  Inputs=+-
  Add6 : Sum
  Constant : Constant  Value=30
  Constant1 : Constant  Value=2
  Constant2 : Constant  Value=0
  Constant3 : Constant  Value=0
  Demux : Demux  Outputs=2
  Divide : Product  Inputs=*/
  Divide1 : Product  Inputs=*/
  Gain : Gain  Gain=8
  Gain1 : Gain  Gain=Rs
  Gain11 : Gain  Gain=bm
  Gain4 : Gain  Gain=Rs
  Gain5 : Gain  Gain=1/J
  Gain7 : Gain  Gain=3*np/(2*k^2)
  Gain9 : Gain  Gain=np
  Integrator : Integrator
  Integrator1 : Integrator
  Integrator2 : Integrator
  Manual Switch : ManualSwitch  CurrentSetting=0
  Mux : Mux  Inputs=3
  Product{,1..6} (7 alike) : Product
  Scope{,1..8} (9 alike) : Scope
  Scope9 : Scope  NumInputPorts=2
  Signal Builder : Subsystem  Tag=STV Subsys  LoadFcn=sigbuilder_block('load');  StartFcn=sigbuilder_block('start');  StopFcn=sigbuilder_block('stop');  ClipboardFcn=sigbuilder_block('clipboard');  mask(Sigbuilder block){tuvar=[0:10]}
      mask help: Simulink:masks:SigbuilderBlock_MD
      mask init:
      | if ~strcmp(get_param(bdroot(gcbh),'SimulationStatus'),'stopped') tuvar = sigbuilder_block('maskInit'); end
      settings: CopyFcn=sigbuilder_block('copy');  DeleteFcn=sigbuilder_block('delete');  ModelCloseFcn=sigbuilder_block('modelClose');  PreSaveFcn=sigbuilder_block('preSave');  PauseFcn=sigbuilder_block('pause');  ContinueFcn=sigbuilder_block('continue');  NameChangeFcn=sigbuilder_block('namechange');  OpenFcn=sigbuilder_block('open',[437.6 199.2 550.4 400 ]);  CloseFcn=sigbuilder_block('close');
      mask Display: plot(0, 0, 100, 100,[2, 2, 32, 32, 2], [68, 8, 8, 68, 68],[32, 2], [38, 38], [32, 19, 2],[53, 60, 44], [32, 17, 17, 2],[16, 16, 31, 31]);txt = getActiveGroup(gcbh);text(2, 100, txt,'verticalAlignment', 'top');
  Unit Delay2 : UnitDelay  SampleTime=-1  HasFrameUpgradeWarning=on
  Unit Delay3 : UnitDelay  SampleTime=-1  HasFrameUpgradeWarning=on
  prevent div by 1 : Subsystem
  prevent div by 2 : Subsystem
  Idq : Outport  VectorParamsAs1DForOutWhenUnconnected=off
  "w_m " : Outport  Port=2  VectorParamsAs1DForOutWhenUnconnected=off
  "Te " : Outport  Port=3  VectorParamsAs1DForOutWhenUnconnected=off
  tag scope: Id=global, Iq=global, Te=global, w_m=global, w_r=global
  wires:
  Add3/1 -> Gain5/1
  Add2/1 -> Product1/1, Scope8/1
  Product5/1 -> Add2/1
  Gain1/1 -> Add/1
  Gain5/1 -> Integrator2/1
  Gain7/1 -> Add3/1, [Te], Scope/1  "Te"
  [psi] -> Product2/2
  Add4/1 -> Gain7/1
  [Iq] -> Product3/1
  Product2/1 -> Add4/1, Scope7/1  "magnet torque"
  [Iq] -> Product2/1
  Product4/1 -> Add/3
  [w_r] -> Product/1
  [Iq] -> Unit Delay3/1
  [w_r] -> Product1/2
  [psi] -> Add2/2
  Gain4/1 -> Add1/1
  Product1/1 -> Add1/3
  Add1/1 -> Divide1/1
  [Ud] -> Add/2
  Add/1 -> Divide/1
  [Uq] -> Add1/2
  [Id] -> Product3/2
  Udq/1 -> Demux/1
  Integrator2/1 -> Gain9/1, [w_m], Scope3/1  "w_m"
  Gain9/1 -> Scope4/1, [w_r]
  [w_m] -> Gain11/1
  [Id] -> Mux/1
  [Iq] -> Mux/2
  [w_m] -> "w_m "/1
  Constant3/1 -> Mux/3
  [Te] -> "Te "/1
  Demux/1 -> Scope9/1, [Ud]
  Demux/2 -> Scope9/2, [Uq]
  Mux/1 -> Idq/1
  psi/1 -> [psi]
  Ld/1 -> [Ld]
  Lq/1 -> [Lq]
  Product/1 -> Product4/1
  [Lq] -> Product4/2
  [Id] -> Unit Delay2/1
  [Ld] -> Product5/1
  [Ld] -> Add5/1
  [Lq] -> Add5/2
  Product3/1 -> Product6/1
  Product6/1 -> Scope5/1, Add4/2
  Add5/1 -> Product6/2
  Integrator1/1 -> [Iq], Gain4/1, Scope2/1
  Integrator/1 -> Scope1/1, Gain1/1, [Id]
  Unit Delay2/1 -> Product5/2
  Unit Delay3/1 -> Product/2
  Divide/1 -> Integrator/1
  Divide1/1 -> Integrator1/1
  Gain11/1 -> Add6/1
  Constant1/1 -> Add6/2
  Signal Builder/1(Signal 1) -> Gain/1
  Gain/1 -> Scope6/1
  [Lq] -> prevent div by 2/1(IN)
  prevent div by 2/1(OUT) -> Divide1/2
  [Ld] -> prevent div by 1/1(IN)
  prevent div by 1/1(OUT) -> Divide/2
  Manual Switch/1 -> Add3/2  "Tload"
  Constant/1 -> Manual Switch/1
  Constant2/1 -> Manual Switch/2

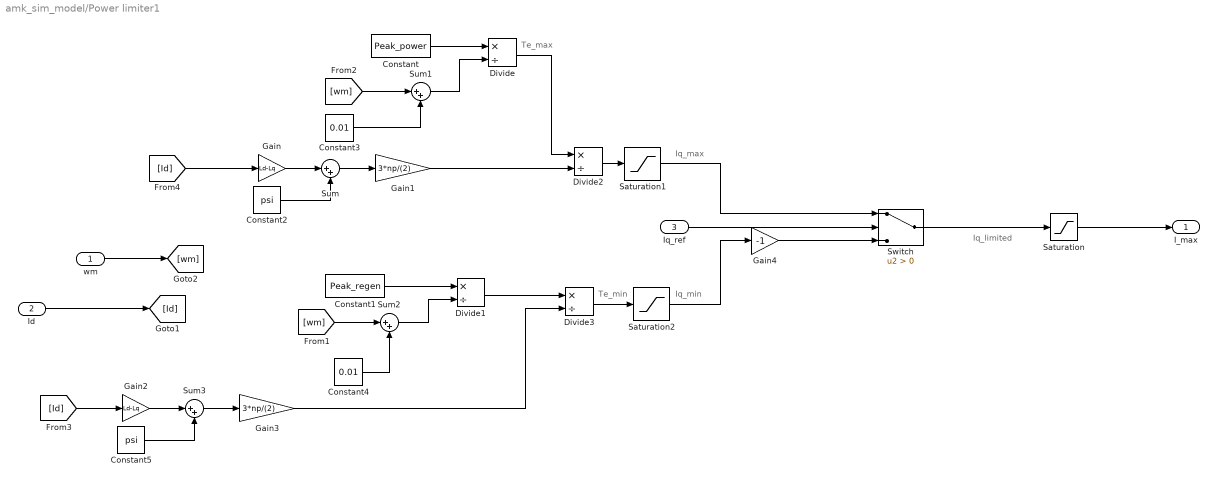
== system amk_sim_model/Power limiter1 ==
  note: Te_max
  note: Iq_limited
  note: Iq_max
  note: Iq_min
  note: Te_min
  wm : Inport
  Id : Inport  Port=2
  Iq_ref : Inport  Port=3
  Constant : Constant  Value=Peak_power
  Constant1 : Constant  Value=Peak_regen
  Constant2 : Constant  Value=psi
  Constant3 : Constant  Value=0.01
  Constant4 : Constant  Value=0.01
  Constant5 : Constant  Value=psi
  Divide{,1..3} (4 alike) : Product  Inputs=*/
  Gain : Gain  Gain=Ld-Lq
  Gain1 : Gain  Gain=3*np/(2)
  Gain2 : Gain  Gain=Ld-Lq
  Gain3 : Gain  Gain=3*np/(2)
  Gain4 : Gain  Gain=-1
  Saturation : Saturate  UpperLimit=I_max  LowerLimit=-I_max
  Saturation1 : Saturate  UpperLimit=10000  LowerLimit=-10000
  Saturation2 : Saturate  UpperLimit=10000  LowerLimit=-10000
  Sum{,1..3} (4 alike) : Sum  Inputs=|++
  Switch : Switch  Criteria=u2 > Threshold  SaturateOnIntegerOverflow=off  InputSameDT=off
  I_max : Outport
  wires:
  Sum2/1 -> Divide1/2
  [wm] -> Sum2/1
  Constant4/1 -> Sum2/2
  Saturation2/1 -> Gain4/1
  Saturation1/1 -> Switch/1
  Constant3/1 -> Sum1/2
  [wm] -> Sum1/1
  Sum1/1 -> Divide/2
  Divide2/1 -> Saturation1/1
  Divide3/1 -> Saturation2/1
  Divide/1 -> Divide2/1
  Constant1/1 -> Divide1/1
  Constant/1 -> Divide/1
  Divide1/1 -> Divide3/1
  Switch/1 -> Saturation/1
  wm/1 -> [wm]
  Iq_ref/1 -> Switch/2
  Gain/1 -> Sum/1
  Constant2/1 -> Sum/2
  Sum/1 -> Gain1/1
  Sum3/1 -> Gain3/1
  [Id] -> Gain2/1
  Gain2/1 -> Sum3/1
  Constant5/1 -> Sum3/2
  [Id] -> Gain/1
  Gain3/1 -> Divide3/2
  Gain1/1 -> Divide2/2
  Id/1 -> [Id]
  Gain4/1 -> Switch/3
  Saturation/1 -> I_max/1

== system amk_sim_model/Signal Builder ==
  Demux : Demux  Tag=STV Demux  Outputs=1
      settings: DisplayOption=none
  FromWs : FromWorkspace  Tag=STV FromWs  VariableName=tuvar
      SigBuilderData=|
      | common.afterFinalStr = 'Extrapolate'
      | common.sampleTime = 0
      | dataSet.timeRange = [0 10]
      | dataSet.name = 'Group 1'
      | sbobj.Groups.Name = 'Group 1'
      | sbobj.Groups.Signals.Name = 'Signal 1'
      | sbobj.Groups.Signals.XData = [0 0.001 0.002 0.003 0.004 0.005 0.006 0.007 0.008 0.009 0.01 0.011 ... (10001 elements, 1x10001)]
      | sbobj.Groups.Signals.YData = [0.537667139546 1.8338850146 -2.258846861 0.862173320368 0.318765239859 -1.30768829631 -0.433592022306 0.342624466539 3.57839693973 2.76943702988 -1.34988694016 3.03492346633 ... (10001 elements, 1x10001)]
  Signal 1 : Outport  Tag=STV Outport
  wires:
  FromWs/1 -> Demux/1
  Demux/1 -> Signal 1/1

== system amk_sim_model/Speed Limiter ==
  note: input
  wm : Inport
  N_max : Inport  Port=2
  I_ref : Inport  Port=3
  Id_Ref : Inport  Port=4
  Iq_Ref : Inport  Port=5
  I_max : Inport  Port=6
  psi : Inport  Port=7
  Constant2 : Constant  Value=0
  Gain4 : Gain  Gain=60/(2*pi)
  Max : MinMax  Function=max  Inputs=2
  Min : MinMax  Inputs=2
  Scope : Scope  NumInputPorts=2
  Sign : Signum
  Switch : Switch  Criteria=u2 > Threshold  SaturateOnIntegerOverflow=off  InputSameDT=off
  speed controller : Subsystem
  speed controller1 : Subsystem
  I_ref_limited : Outport
  wires:
  speed controller1/1(Iq_ref) -> Max/2
  Max/1 -> Switch/3
  I_ref/1 -> Max/1, Sign/1, Scope/2, Min/2
  [Iq_ref] -> speed controller/4(Iq_ref_sat)
  [Id_ref] -> speed controller/3(Id_ref)
  speed controller/1(Iq_ref) -> Scope/1, Min/1
  Gain4/1 -> speed controller1/2(N), speed controller/2(N)
  N_max/1 -> speed controller/1(N_ref)
  Constant2/1 -> speed controller1/1(N_ref)
  Min/1 -> Switch/1
  Sign/1 -> Switch/2
  wm/1 -> Gain4/1
  Switch/1 -> I_ref_limited/1
  Iq_Ref/1 -> [Iq_ref]
  I_max/1 -> [I_max]
  [I_max] -> speed controller1/5(I_max)
  [I_max] -> speed controller/5(I_max)
  [psi] -> speed controller/6(psi)
  [Id_ref] -> speed controller1/3(Id_ref)
  [Iq_ref] -> speed controller1/4(Iq_ref_sat)
  [psi] -> speed controller1/6(psi)
  psi/1 -> [psi]
  Id_Ref/1 -> [Id_ref]

== system amk_sim_model/Subsystem ==
  ramp1 : Inport
  ramp2 : Inport  Port=2
  sampling time : Inport  Port=3
  rise time (Amp/ms) : Inport  Port=4
  Constant5 : Constant  Value=0
  Gain : Gain  Gain=1000
  Gain1 : Gain  Gain=0.1
  Memory1 : Memory
  Memory2 : Memory
  Product : Product
  Product1 : Product
  Saturation Dynamic1 : simulink/Discontinuities/Saturation Dynamic  OutMin=[]  OutMax=[]  OutDataTypeStr=Inherit: Same as second input  OutDataType=fixdt(1, 16)  OutScaling=2^-10  DoSatur=off
  Step3 : Step  Time=0.25  Before=1  After=-1  SampleTime=0
  Sum1 : Sum  Inputs=|+++
  Sum4 : Sum  Inputs=|-+
  Switch1 : Switch  Criteria=u2 > Threshold  SaturateOnIntegerOverflow=off  InputSameDT=off
  Switch2 : Switch  Criteria=u2 > Threshold  SaturateOnIntegerOverflow=off  InputSameDT=off
  I_ramped : Outport
  wires:
  Sum1/1 -> Memory2/1, Sum4/1, Memory1/1, Saturation Dynamic1/2
  Switch2/1 -> Product1/2
  Memory2/1 -> Switch2/2
  Product1/1 -> Sum1/1
  Memory1/1 -> Sum1/3
  Gain1/1 -> Switch2/3
  Switch1/1 -> Saturation Dynamic1/3
  Step3/1 -> Switch1/2, Product1/1  "Id*"
  Sum4/1 -> Sum1/2
  Constant5/1 -> Switch1/1
  Saturation Dynamic1/1 -> Sum4/2, I_ramped/1
  ramp2/1 -> Switch1/3
  ramp1/1 -> Saturation Dynamic1/1
  rise time (Amp/ms)/1 -> Gain/1
  sampling time/1 -> Product/2
  Gain/1 -> Product/1
  Product/1 -> Switch2/1, Gain1/1

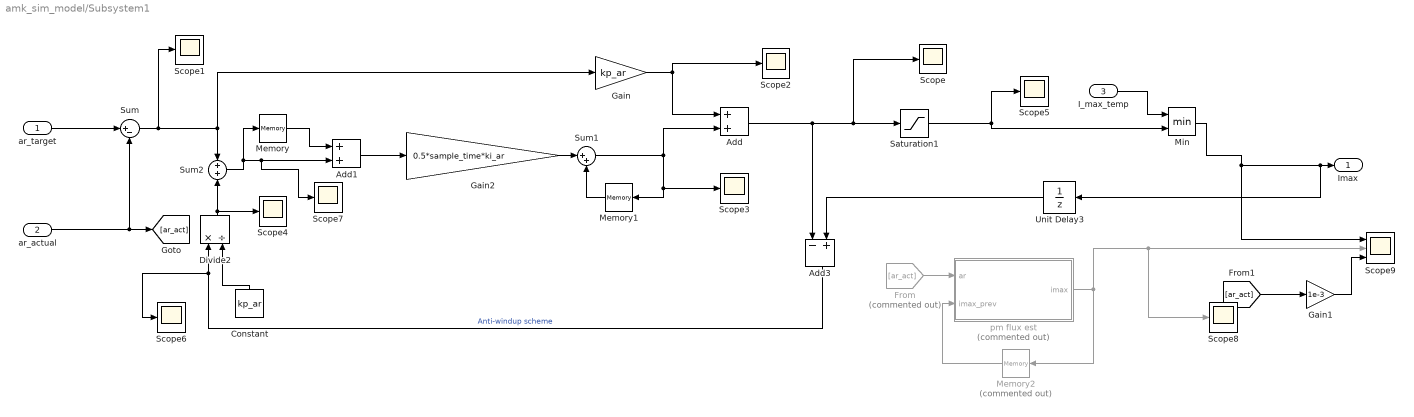
== system amk_sim_model/Subsystem1 ==
  ar_target : Inport
  ar_actual : Inport  Port=2
  I_max_temp : Inport  Port=3
  Add : Sum
  Add1 : Sum
  Add3 : Sum  Inputs=-+
  Constant : Constant  Value=kp_ar
  Divide2 : Product  Inputs=*/
  From : From  Commented=on  GotoTag=ar_act
  Gain : Gain  Gain=kp_ar
  Gain1 : Gain  Gain=1e-3
  Gain2 : Gain  Gain=0.5*sample_time*ki_ar
  Memory : Memory
  Memory1 : Memory
  Memory2 : Memory  Commented=on
  Min : MinMax  Inputs=2
  Saturation1 : Saturate  UpperLimit=I_max  LowerLimit=0
  Scope{,1..8} (9 alike) : Scope
  Scope9 : Scope  NumInputPorts=3
  Sum : Sum  Inputs=|+-
  Sum1 : Sum  Inputs=|++
  Sum2 : Sum
  Unit Delay3 : UnitDelay  SampleTime=-1  HasFrameUpgradeWarning=on
  pm flux est : MATLAB Function  Commented=on  TreatAsAtomicUnit=on
  Imax : Outport
  wires:
  ar_target/1 -> Sum/1
  Sum/1 -> Scope1/1, Sum2/1, Gain/1
  Gain/1 -> Add/1, Scope2/1
  Divide2/1 -> Sum2/2, Scope4/1
  Constant/1 -> Divide2/2
  Add3/1 -> Divide2/1, Scope6/1  "Anti-windup scheme"
  Add/1 -> Saturation1/1, Scope/1, Add3/1
  Unit Delay3/1 -> Add3/2
  Saturation1/1 -> Scope5/1, Min/2
  I_max_temp/1 -> Min/1
  Sum2/1 -> Scope7/1, Add1/2, Memory/1
  Add1/1 -> Gain2/1
  Memory/1 -> Add1/1
  Gain2/1 -> Sum1/1
  Memory1/1 -> Sum1/2
  Sum1/1 -> Add/2, Scope3/1, Memory1/1
  ar_actual/1 -> [ar_act], Sum/2
  From/1 -> pm flux est/1(ar)
  pm flux est/1(imax) -> Memory2/1, Scope8/1, Scope9/2
  Memory2/1 -> pm flux est/2(imax_prev)
  Min/1 -> Unit Delay3/1, Imax/1, Scope9/1
  Gain1/1 -> Scope9/3
  [ar_act] -> Gain1/1

== system amk_sim_model/Subsystem2 ==
  temp : Inport
  max_temp : Inport  Port=2
  derate_threshold : Inport  Port=3
  Add : Sum  Inputs=+-
  Add1 : Sum  Inputs=+-
  Add2 : Sum  Inputs=+-
  Constant : Constant  Value=I_max
  Divide : Product  Inputs=*/
  Product : Product
  Saturation : Saturate  UpperLimit=1000  LowerLimit=0
  Scope : Scope  NumInputPorts=2
  Square : Math  Operator=square
  I_max : Outport
  wires:
  max_temp/1 -> Add/1
  Add/1 -> [distance]
  derate_threshold/1 -> [derate_threshold], Add/2
  [derate_threshold] -> Add1/2
  temp/1 -> Add1/1
  Add1/1 -> Saturation/1
  Saturation/1 -> [diff]
  [distance] -> Add2/1
  [diff] -> Add2/2
  Add2/1 -> Divide/1
  [distance] -> Divide/2
  Divide/1 -> Square/1
  Constant/1 -> Product/2, Scope/2
  Square/1 -> Product/1
  Product/1 -> Scope/1, I_max/1

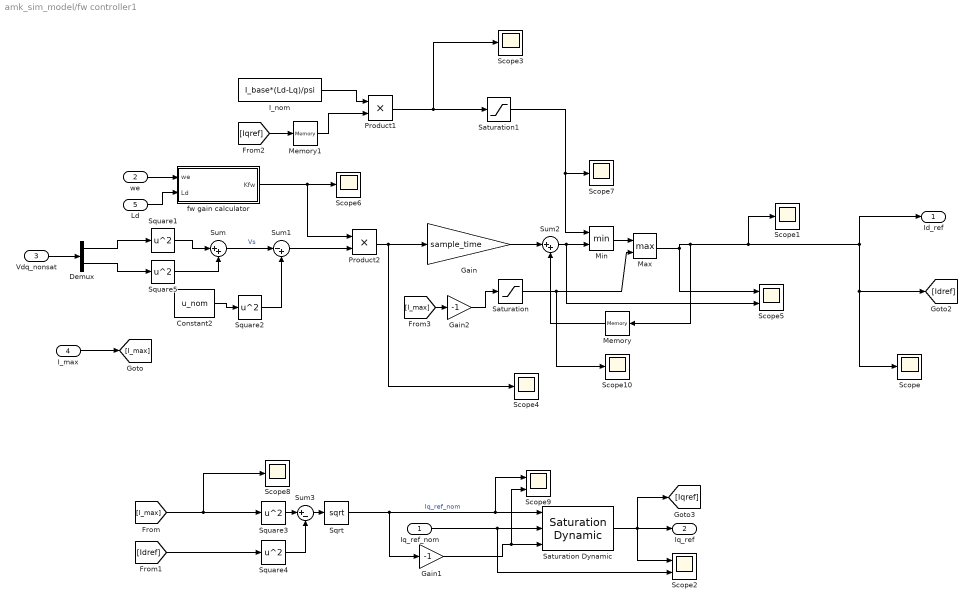
== system amk_sim_model/fw controller1 ==
  Iq_ref_nom : Inport
  we : Inport  Port=2
  Vdq_nonsat : Inport  Port=3
  I_max : Inport  Port=4
  Ld : Inport  Port=5
  Constant2 : Constant  Value=u_nom
  Demux : Demux  Outputs=2
  Gain : Gain  Gain=sample_time
  Gain1 : Gain  Gain=-1
  Gain2 : Gain  Gain=-1
  I_nom : Constant  Value=I_base*(Ld-Lq)/psi
  Max : MinMax  Function=max  Inputs=2
  Memory : Memory
  Memory1 : Memory
  Min : MinMax  Inputs=2
  Product1 : Product
  Product2 : Product
  Saturation : Saturate  UpperLimit=-50  LowerLimit=-200
  Saturation Dynamic : simulink/Discontinuities/Saturation Dynamic  OutMin=[]  OutMax=[]  OutDataTypeStr=Inherit: Same as second input  OutDataType=fixdt(1, 16)  OutScaling=2^-10  DoSatur=off
  Saturation1 : Saturate  UpperLimit=20  LowerLimit=-20
  Scope{,1,3..4,6..8,10} (8 alike) : Scope
  Scope2 : Scope  NumInputPorts=2
  Scope5 : Scope  NumInputPorts=2
  Scope9 : Scope  NumInputPorts=2
  Sqrt : Sqrt
  Square{1..5} (5 alike) : Math  Operator=square
  Sum : Sum  Inputs=|++
  Sum1 : Sum  Inputs=|-+
  Sum2 : Sum  Inputs=|++
  Sum3 : Sum  Inputs=|+-
  fw gain calculator : Subsystem
  Id_ref : Outport
  Iq_ref : Outport  Port=2
  wires:
  Max/1 -> Scope5/1, Memory/1, Scope1/1, [Idref], Scope/1, Id_ref/1
  Product2/1 -> Scope4/1, Gain/1
  Sum1/1 -> Product2/2
  fw gain calculator/1(Kfw) -> Scope6/1, Product2/1
  [Iqref] -> Memory1/1
  Square5/1 -> Sum/2
  Square1/1 -> Sum/1
  Vdq_nonsat/1 -> Demux/1
  Demux/1 -> Square1/1
  Demux/2 -> Square5/1
  I_nom/1 -> Product1/1
  Gain1/1 -> Scope9/2, Saturation Dynamic/3
  Sum3/1 -> Sqrt/1
  Constant2/1 -> Square2/1
  Sum/1 -> Sum1/1  "Vs"
  Square2/1 -> Sum1/2
  we/1 -> fw gain calculator/1(we)
  Square3/1 -> Sum3/1
  Square4/1 -> Sum3/2
  Sqrt/1 -> Scope9/1, Saturation Dynamic/1, Gain1/1  "Iq_ref_nom"
  Saturation Dynamic/1 -> Scope2/1, Iq_ref/1, [Iqref]
  Gain/1 -> Sum2/1
  Sum2/1 -> Min/2, Scope5/2
  Memory/1 -> Sum2/2
  Product1/1 -> Saturation1/1, Scope3/1
  Gain2/1 -> Saturation/1
  Min/1 -> Max/1
  Saturation/1 -> Scope10/1, Max/2
  Saturation1/1 -> Min/1, Scope7/1
  Memory1/1 -> Product1/2
  I_max/1 -> [I_max]
  [I_max] -> Gain2/1
  [I_max] -> Scope8/1, Square3/1
  Iq_ref_nom/1 -> Scope2/2, Saturation Dynamic/2
  [Idref] -> Square4/1
  Ld/1 -> fw gain calculator/2(Ld)

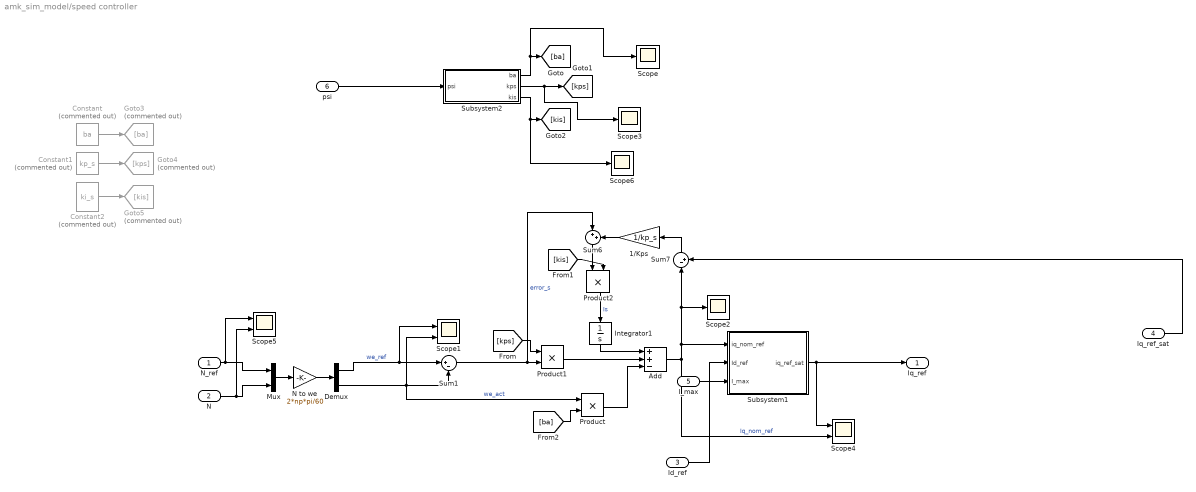
== system amk_sim_model/speed controller ==
  N_ref : Inport
  N : Inport  Port=2
  Id_ref : Inport  Port=3
  Iq_ref_sat : Inport  Port=4
  I_max : Inport  Port=5
  psi : Inport  Port=6
  1/Kps : Gain  Gain=1/kp_s
  Add : Sum  Inputs=++-
  Constant : Constant  Commented=on  Value=ba
  Constant1 : Constant  Commented=on  Value=kp_s
  Constant2 : Constant  Commented=on  Value=ki_s
  Demux : Demux  Outputs=2
  Goto3 : Goto  Commented=on  GotoTag=ba
  Goto4 : Goto  Commented=on  GotoTag=kps
  Goto5 : Goto  Commented=on  GotoTag=kis
  Integrator1 : Integrator
  Mux : Mux  Inputs=2
  N to we : Gain  Gain=2*np*pi/60
  Product : Product
  Product1 : Product
  Product2 : Product
  Scope{,2..3,6} (4 alike) : Scope
  Scope1 : Scope  NumInputPorts=2
  Scope4 : Scope  NumInputPorts=2
  Scope5 : Scope  NumInputPorts=2
  Subsystem1 : Subsystem
  Subsystem2 : Subsystem
  Sum1 : Sum  Inputs=|+-
  Sum6 : Sum  Inputs=|++
  Sum7 : Sum  Inputs=|-+
  Iq_ref : Outport
  wires:
  Sum7/1 -> 1/Kps/1
  Add/1 -> Scope2/1, Sum7/1, Subsystem1/1(iq_nom_ref), Scope4/2  "Iq_nom_ref"
  Product1/1 -> Add/2
  1/Kps/1 -> Sum6/2
  Sum1/1 -> Product1/2, Sum6/1  "error_s"
  N_ref/1 -> Scope5/1, Mux/1
  N/1 -> Scope5/2, Mux/2
  [ba] -> Product/2
  Product2/1 -> Integrator1/1  "Is"
  Product/1 -> Add/3
  Demux/1 -> Scope1/1, Sum1/1  "we_ref"
  Demux/2 -> Product/1, Sum1/2, Scope1/2  "we_act"
  Sum6/1 -> Product2/1
  Subsystem1/1(iq_ref_sat) -> Scope4/1, Iq_ref/1
  Mux/1 -> N to we/1
  N to we/1 -> Demux/1
  Integrator1/1 -> Add/1
  Id_ref/1 -> Subsystem1/2(Id_ref)
  I_max/1 -> Subsystem1/3(I_max)
  psi/1 -> Subsystem2/1(psi)
  Subsystem2/1(ba) -> Scope/1, [ba]
  Subsystem2/2(kps) -> Scope3/1, [kps]
  Subsystem2/3(kis) -> Scope6/1, [kis]
  [kps] -> Product1/1
  [kis] -> Product2/2
  Constant/1 -> Goto3/1
  Constant1/1 -> Goto4/1
  Constant2/1 -> Goto5/1
  Iq_ref_sat/1 -> Sum7/2

== system amk_sim_model/Current Controller/Signal Builder ==
  Demux : Demux  Tag=STV Demux  Outputs=1
      settings: DisplayOption=none
  FromWs : FromWorkspace  Tag=STV FromWs  VariableName=tuvar
      SigBuilderData=|
      | common.afterFinalStr = 'Extrapolate'
      | common.sampleTime = 0
      | dataSet.timeRange = [0 10]
      | dataSet.name = 'Group 1'
      | sbobj.Groups.Name = 'Group 1'
      | sbobj.Groups.Signals.Name = 'Signal 2'
      | sbobj.Groups.Signals.XData = [0 0.01 0.02 0.03 0.04 0.05 0.06 0.07 0.08 0.09 0.1 0.11 ... (1001 elements, 1x1001)]
      | sbobj.Groups.Signals.YData = [-0.131067824281 -0.768631666817 2.38995183631 0.0772456795913 0.375607450233 0.395564169368 -0.11249908896 -1.82903670222 2.09145219348 0.359093122201 -0.794344747027 -0.227311640661 ... (1001 elements, 1x1001)]
  Signal 2 : Outport  Tag=STV Outport
  wires:
  FromWs/1 -> Demux/1
  Demux/1 -> Signal 2/1

== system amk_sim_model/Current Controller/Signal Builder1 ==
  Demux : Demux  Tag=STV Demux  Outputs=1
      settings: DisplayOption=none
  FromWs : FromWorkspace  Tag=STV FromWs  VariableName=tuvar
      SigBuilderData=|
      | common.afterFinalStr = 'Extrapolate'
      | common.sampleTime = 0
      | dataSet.timeRange = [0 10]
      | dataSet.name = 'Group 1'
      | sbobj.Groups.Name = 'Group 1'
      | sbobj.Groups.Signals.Name = 'Signal 2'
      | sbobj.Groups.Signals.XData = [0 0.01 0.02 0.03 0.04 0.05 0.06 0.07 0.08 0.09 0.1 0.11 ... (1001 elements, 1x1001)]
      | sbobj.Groups.Signals.YData = [-0.131067824281 -0.768631666817 2.38995183631 0.0772456795913 0.375607450233 0.395564169368 -0.11249908896 -1.82903670222 2.09145219348 0.359093122201 -0.794344747027 -0.227311640661 ... (1001 elements, 1x1001)]
  Signal 2 : Outport  Tag=STV Outport
  wires:
  Demux/1 -> Signal 2/1
  FromWs/1 -> Demux/1

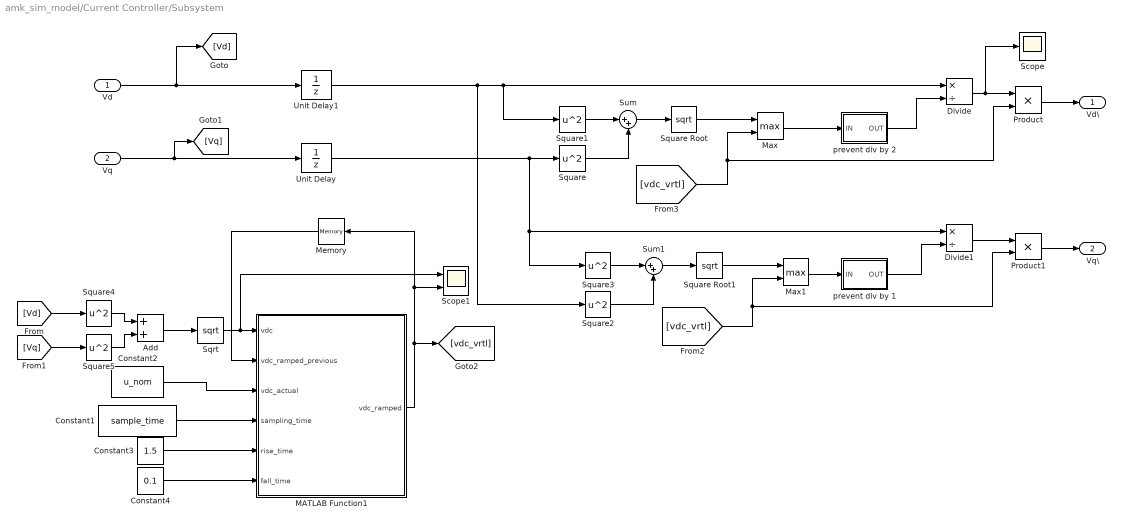
== system amk_sim_model/Current Controller/Subsystem ==
  Vd : Inport
  Vq : Inport  Port=2
  Add : Sum
  Constant1 : Constant  Value=sample_time
  Constant2 : Constant  Value=u_nom
  Constant3 : Constant  Value=1.5
  Constant4 : Constant  Value=0.1
  Divide : Product  Inputs=*/
  Divide1 : Product  Inputs=*/
  MATLAB Function1 : MATLAB Function  TreatAsAtomicUnit=on
  Max : MinMax  Function=max  Inputs=2
  Max1 : MinMax  Function=max  Inputs=2
  Memory : Memory
  Product : Product
  Product1 : Product
  Scope : Scope
  Scope1 : Scope  NumInputPorts=2
  Sqrt : Sqrt
  Square{,1..5} (6 alike) : Math  Operator=square
  Square Root : Sqrt
  Square Root1 : Sqrt
  Sum : Sum  Inputs=|++
  Sum1 : Sum  Inputs=|++
  Unit Delay : UnitDelay  SampleTime=-1  HasFrameUpgradeWarning=on
  Unit Delay1 : UnitDelay  SampleTime=-1  HasFrameUpgradeWarning=on
  prevent div by 1 : Subsystem
  prevent div by 2 : Subsystem
  Vd\ : Outport
  Vq\ : Outport  Port=2
  wires:
  Square1/1 -> Sum/1
  Square/1 -> Sum/2
  Sum/1 -> Square Root/1
  Square Root/1 -> Max/1
  [vdc_vrtl] -> Product/2, Max/2
  Max/1 -> prevent div by 2/1(IN)
  Divide/1 -> Scope/1, Product/1
  Product/1 -> Vd\/1
  Square3/1 -> Sum1/1
  [vdc_vrtl] -> Product1/2, Max1/2
  Square2/1 -> Sum1/2
  Divide1/1 -> Product1/1
  Vd/1 -> [Vd], Unit Delay1/1
  Vq/1 -> [Vq], Unit Delay/1
  Square Root1/1 -> Max1/1
  Max1/1 -> prevent div by 1/1(IN)
  Sum1/1 -> Square Root1/1
  Product1/1 -> Vq\/1
  [Vd] -> Square4/1
  [Vq] -> Square5/1
  Square4/1 -> Add/1
  Square5/1 -> Add/2
  Add/1 -> Sqrt/1
  Sqrt/1 -> Scope1/1, MATLAB Function1/1(vdc)
  Memory/1 -> MATLAB Function1/2(vdc_ramped_previous)
  MATLAB Function1/1(vdc_ramped) -> [vdc_vrtl], Memory/1, Scope1/2
  Constant2/1 -> MATLAB Function1/3(vdc_actual)
  Unit Delay/1 -> Divide1/1, Square3/1, Square/1
  Unit Delay1/1 -> Square2/1, Divide/1, Square1/1
  prevent div by 2/1(OUT) -> Divide/2
  prevent div by 1/1(OUT) -> Divide1/2
  Constant1/1 -> MATLAB Function1/4(sampling_time)
  Constant3/1 -> MATLAB Function1/5(rise_time)
  Constant4/1 -> MATLAB Function1/6(fall_time)

== system amk_sim_model/Current Controller/Subsystem1 ==
  Vd : Inport
  Vq : Inport  Port=2
  Constant : Constant  Value=u_nom
  Constant1 : Constant  Value=u_nom
  Divide : Product  Inputs=*/
  Divide1 : Product  Inputs=*/
  Max : MinMax  Function=max  Inputs=2
  Max1 : MinMax  Function=max  Inputs=2
  Product : Product
  Product1 : Product
  Scope : Scope
  Square{,1..3} (4 alike) : Math  Operator=square
  Square Root : Sqrt
  Square Root1 : Sqrt
  Sum : Sum  Inputs=|++
  Sum1 : Sum  Inputs=|++
  Unit Delay : UnitDelay  SampleTime=-1  HasFrameUpgradeWarning=on
  Unit Delay1 : UnitDelay  SampleTime=-1  HasFrameUpgradeWarning=on
  prevent div by 1 : Subsystem
  prevent div by 2 : Subsystem
  Vd\ : Outport
  Vq\ : Outport  Port=2
  wires:
  Square1/1 -> Sum/1
  Square/1 -> Sum/2
  Sum/1 -> Square Root/1
  Square Root/1 -> Max/1
  Constant1/1 -> Product/2, Max/2
  Max/1 -> prevent div by 2/1(IN)
  Divide/1 -> Scope/1, Product/1
  Product/1 -> Vd\/1
  Square3/1 -> Sum1/1
  Constant/1 -> Product1/2, Max1/2
  Square2/1 -> Sum1/2
  Divide1/1 -> Product1/1
  Vd/1 -> Unit Delay1/1
  Vq/1 -> Unit Delay/1
  Square Root1/1 -> Max1/1
  Max1/1 -> prevent div by 1/1(IN)
  Sum1/1 -> Square Root1/1
  Product1/1 -> Vq\/1
  Unit Delay/1 -> Divide1/1, Square3/1, Square/1
  Unit Delay1/1 -> Square2/1, Divide/1, Square1/1
  prevent div by 2/1(OUT) -> Divide/2
  prevent div by 1/1(OUT) -> Divide1/2

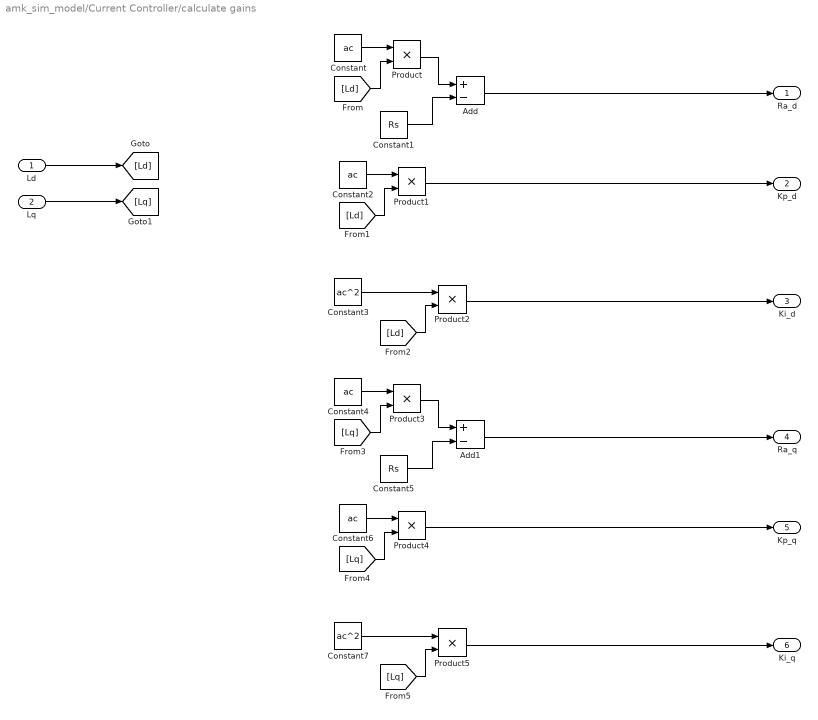
== system amk_sim_model/Current Controller/calculate gains ==
  Ld : Inport
  Lq : Inport  Port=2
  Add : Sum  Inputs=+-
  Add1 : Sum  Inputs=+-
  Constant{,2,4,6} (4 alike) : Constant  Value=ac
  Constant1 : Constant  Value=Rs
  Constant3 : Constant  Value=ac^2
  Constant5 : Constant  Value=Rs
  Constant7 : Constant  Value=ac^2
  Product{,1..5} (6 alike) : Product
  Ra_d : Outport
  Kp_d : Outport  Port=2
  Ki_d : Outport  Port=3
  Ra_q : Outport  Port=4
  Kp_q : Outport  Port=5
  Ki_q : Outport  Port=6
  wires:
  Constant/1 -> Product/1
  Ld/1 -> [Ld]
  Lq/1 -> [Lq]
  [Ld] -> Product/2
  Constant1/1 -> Add/2
  Product/1 -> Add/1
  Add/1 -> Ra_d/1
  Product1/1 -> Kp_d/1
  [Ld] -> Product1/2
  Constant2/1 -> Product1/1
  Constant3/1 -> Product2/1
  [Ld] -> Product2/2
  Product2/1 -> Ki_d/1
  Product5/1 -> Ki_q/1
  [Lq] -> Product5/2
  Constant7/1 -> Product5/1
  Constant6/1 -> Product4/1
  [Lq] -> Product4/2
  Product4/1 -> Kp_q/1
  Add1/1 -> Ra_q/1
  Product3/1 -> Add1/1
  Constant5/1 -> Add1/2
  [Lq] -> Product3/2
  Constant4/1 -> Product3/1

== system amk_sim_model/I2t/prevent div by 0 ==
  IN : Inport
  Constant : Constant  Value=0.0001
  Switch : Switch  Criteria=u2 > Threshold  Threshold=0.0001  SaturateOnIntegerOverflow=off  InputSameDT=off  OutDataTypeStr=Inherit: Same as first input
  OUT : Outport  VectorParamsAs1DForOutWhenUnconnected=off
  wires:
  IN/1 -> Switch/2, Switch/1
  Switch/1 -> OUT/1
  Constant/1 -> Switch/3

== system amk_sim_model/I2t/prevent div by 1 ==
  IN : Inport
  Constant : Constant  Value=0.0001
  Switch : Switch  Criteria=u2 > Threshold  Threshold=0.0001  SaturateOnIntegerOverflow=off  InputSameDT=off  OutDataTypeStr=Inherit: Same as first input
  OUT : Outport  VectorParamsAs1DForOutWhenUnconnected=off
  wires:
  Constant/1 -> Switch/3
  Switch/1 -> OUT/1
  IN/1 -> Switch/1, Switch/2

== system amk_sim_model/I2t/prevent div by 2 ==
  IN : Inport
  Constant : Constant  Value=0.0001
  Switch : Switch  Criteria=u2 > Threshold  Threshold=0.0001  SaturateOnIntegerOverflow=off  InputSameDT=off  OutDataTypeStr=Inherit: Same as first input
  OUT : Outport  VectorParamsAs1DForOutWhenUnconnected=off
  wires:
  Constant/1 -> Switch/3
  Switch/1 -> OUT/1
  IN/1 -> Switch/1, Switch/2

== system amk_sim_model/PMSM signal model/Signal Builder ==
  Demux : Demux  Tag=STV Demux  Outputs=1
      settings: DisplayOption=none
  FromWs : FromWorkspace  Tag=STV FromWs  VariableName=tuvar
      SigBuilderData=|
      | common.afterFinalStr = 'Extrapolate'
      | common.sampleTime = 0
      | dataSet.timeRange = [0 5]
      | dataSet.name = 'Group 1'
      | sbobj.Groups.Name = 'Group 1'
      | sbobj.Groups.Signals.Name = 'Signal 1'
      | sbobj.Groups.Signals.XData = [0 0.05 0.05 0.1 0.1 0.15 0.15 0.2 0.2 0.25 0.25 0.3 0.3 0.35 0.35 0.4 0.4 0.45 0.45 0.5 0.5 0.55 0.55 0.6 0.6 0.65 0.65 0.7 0.7 0.75 0.75 0.8 0.8 0.85 0.85 0.9 0.9 0.95 0.95 1 1 1.05 1.05 1.1 1.1 1.15 1.15 1.2 1.2 1.25 1.25 1.3 1.3 1.35 1.35 1.4 1.4 1.45 1.45 1.5 1.5 1.55 1.55 1.6 1.6 1.65 1.65 1.7 1.7 1.75 1.75 1.8 1.8 1.85 1.85 1.9 1.9 1.95 1.95 2 2 2.05 2.05 2.1 2.1 2.15 2.15 2.2 2.2 2.25 2.25 2.3 2.3 2.35 2.35 2.4 2.4 2.45 2.45 2.5 2.5 2.55 2.55 2.6 2.6 2.65 2.65 2.7 2.7 2.75 2.75 2.8 2.8 2.85 2.85 2.9 2.9 2.95 2.95 3 3 3.05 3.05 3.1 3.1 3.15 3.15 3.2 3.2 3.25 3.25 3.3 3.3 3.35 3.35 3.4 3.4 3.45 3.45 3.5 3.5 3.55 3.55 3.6 3.6 3.65 3.65 3.7 3.7 3.75 3.75 3.8 3.8 3.85 3.85 3.9 3.9 3.95 3.95 4 4 4.05 4.05 4.1 4.1 4.15 4.15 4.2 4.2 4.25 4.25 4.3 4.3 4.35 4.35 4.4 4.4 4.45 4.45 4.5 4.5 4.55 4.55 4.6 4.6 4.65 4.65 4.7 4.7 4.75 4.75 4.8 4.8 4.85 4.85 4.9 4.9 4.95 4.95 5]
      | sbobj.Groups.Signals.YData = [2 2 0 0 2 2 0 0 2 2 0 0 2 2 0 0 2 2 0 0 2 2 0 0 2 2 0 0 2 2 0 0 2 2 0 0 2 2 0 0 2 2 0 0 2 2 0 0 2 2 0 0 2 2 0 0 2 2 0 0 2 2 0 0 2 2 0 0 2 2 0 0 2 2 0 0 2 2 0 0 2 2 0 0 2 2 0 0 2 2 0 0 2 2 0 0 2 2 0 0 2 2 0 0 2 2 0 0 2 2 0 0 2 2 0 0 2 2 0 0 2 2 0 0 2 2 0 0 2 2 0 0 2 2 0 0 2 2 0 0 2 2 0 0 2 2 0 0 2 2 0 0 2 2 0 0 2 2 0 0 2 2 0 0 2 2 0 0 2 2 0 0 2 2 0 0 2 2 0 0 2 2 0 0 2 2 0 0 2 2 0 0 2 2 0 0 2 2 0 0]
      | sbobj.Groups.TimeRange = [0 5]
  Signal 1 : Outport  Tag=STV Outport
  wires:
  FromWs/1 -> Demux/1
  Demux/1 -> Signal 1/1

== system amk_sim_model/PMSM signal model/prevent div by 1 ==
  IN : Inport
  Constant : Constant  Value=0.00001
  Switch : Switch  Criteria=u2 > Threshold  Threshold=0.00001  SaturateOnIntegerOverflow=off  InputSameDT=off  OutDataTypeStr=Inherit: Same as first input
  OUT : Outport  VectorParamsAs1DForOutWhenUnconnected=off
  wires:
  IN/1 -> Switch/2, Switch/1
  Switch/1 -> OUT/1
  Constant/1 -> Switch/3

== system amk_sim_model/PMSM signal model/prevent div by 2 ==
  IN : Inport
  Constant : Constant  Value=0.00001
  Switch : Switch  Criteria=u2 > Threshold  Threshold=0.00001  SaturateOnIntegerOverflow=off  InputSameDT=off  OutDataTypeStr=Inherit: Same as first input
  OUT : Outport  VectorParamsAs1DForOutWhenUnconnected=off
  wires:
  Constant/1 -> Switch/3
  Switch/1 -> OUT/1
  IN/1 -> Switch/1, Switch/2

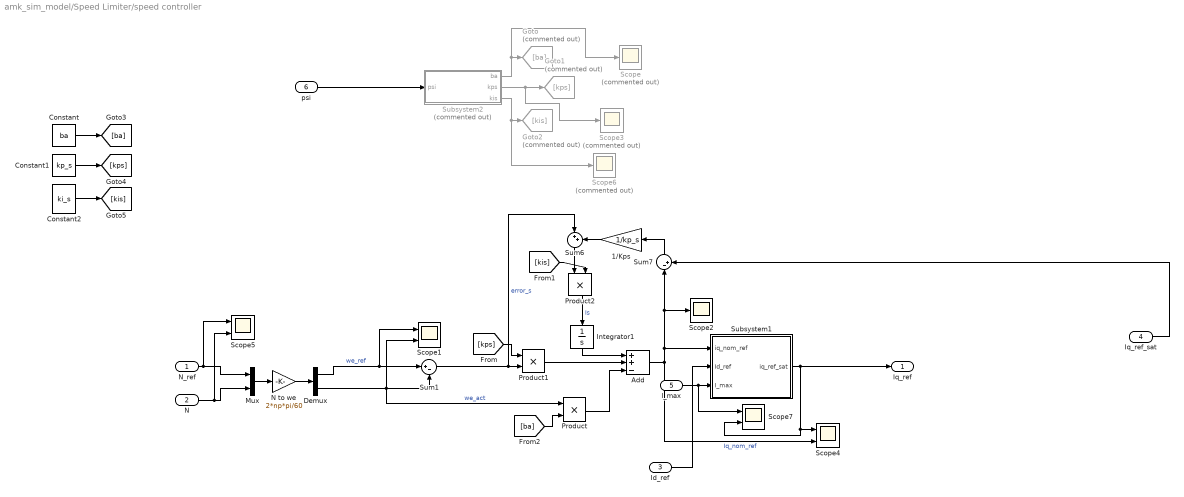
== system amk_sim_model/Speed Limiter/speed controller ==
  N_ref : Inport
  N : Inport  Port=2
  Id_ref : Inport  Port=3
  Iq_ref_sat : Inport  Port=4
  I_max : Inport  Port=5
  psi : Inport  Port=6
  1/Kps : Gain  Gain=1/kp_s
  Add : Sum  Inputs=++-
  Constant : Constant  Value=ba
  Constant1 : Constant  Value=kp_s
  Constant2 : Constant  Value=ki_s
  Demux : Demux  Outputs=2
  Goto : Goto  Commented=on  GotoTag=ba
  Goto1 : Goto  Commented=on  GotoTag=kps
  Goto2 : Goto  Commented=on  GotoTag=kis
  Integrator1 : Integrator
  Mux : Mux  Inputs=2
  N to we : Gain  Gain=2*np*pi/60
  Product : Product
  Product1 : Product
  Product2 : Product
  Scope : Scope  Commented=on
  Scope{1,4..5,7} (4 alike) : Scope  NumInputPorts=2
  Scope2 : Scope
  Scope3 : Scope  Commented=on
  Scope6 : Scope  Commented=on
  Subsystem1 : Subsystem
  Subsystem2 : Subsystem  Commented=on
  Sum1 : Sum  Inputs=|+-
  Sum6 : Sum  Inputs=|++
  Sum7 : Sum  Inputs=|-+
  Iq_ref : Outport
  wires:
  Sum7/1 -> 1/Kps/1
  Add/1 -> Scope2/1, Sum7/1, Subsystem1/1(iq_nom_ref), Scope4/2  "Iq_nom_ref"
  Product1/1 -> Add/2
  1/Kps/1 -> Sum6/2
  Sum1/1 -> Product1/2, Sum6/1  "error_s"
  N_ref/1 -> Scope5/1, Mux/1
  N/1 -> Scope5/2, Mux/2
  [ba] -> Product/2
  Product2/1 -> Integrator1/1  "Is"
  Product/1 -> Add/3
  Demux/1 -> Scope1/1, Sum1/1  "we_ref"
  Demux/2 -> Product/1, Sum1/2, Scope1/2  "we_act"
  Sum6/1 -> Product2/1
  Subsystem1/1(iq_ref_sat) -> Scope7/2, Scope4/1, Iq_ref/1
  Mux/1 -> N to we/1
  N to we/1 -> Demux/1
  Integrator1/1 -> Add/1
  Id_ref/1 -> Subsystem1/2(Id_ref)
  Iq_ref_sat/1 -> Sum7/2
  I_max/1 -> Scope7/1, Subsystem1/3(I_max)
  psi/1 -> Subsystem2/1(psi)
  Subsystem2/1(ba) -> Scope/1, Goto/1
  Subsystem2/2(kps) -> Scope3/1, Goto1/1
  Subsystem2/3(kis) -> Scope6/1, Goto2/1
  [kps] -> Product1/1
  [kis] -> Product2/2
  Constant/1 -> [ba]
  Constant1/1 -> [kps]
  Constant2/1 -> [kis]
